simulink model "MassSpringDamper_Simulink_Model"  (R2023b)
settings: Solver=ode45  StartTime=0.0  StopTime=30  MaxStep=0.01  RelTol=1e-3  EnableMultiTasking=on
model workspace (MAT data in the model file):
  c = 1
  k = 2
  m = 3
settings Model: Creator=The MathWorks, Inc.  LastModifiedBy=AmitW
settings SolverCC: AlgebraicLoopSolver=TrustRegion
settings DataIOCC: LimitDataPoints=on  SaveFormat=Array  SaveOutput=off  SignalLogging=off  SaveTime=off  ReturnWorkspaceOutputs=off
settings OptimizationCC: LifeSpan=inf
settings DebuggingCC: UnconnectedInputMsg=warning  UnconnectedOutputMsg=warning  UnconnectedLineMsg=warning  AllowSymbolicDim=off  SFUnexpectedBacktrackingDiag=warning  SFNoUnconditionalDefaultTransitionDiag=warning  SFExecutionAtInitializationDiag=none  ArithmeticOperatorsInVariantConditions=warning
settings HardwareCC: ProdBitPerPointer=32  ProdBitPerSizeT=32  ProdBitPerPtrDiffT=32  ProdLargestAtomicFloat=None  ProdIntDivRoundTo=Undefined  ProdEndianess=Unspecified  ProdWordSize=32  ProdHWDeviceType=32-bit Generic
settings ModelReferenceCC: EnableRefExpFcnMdlSchedulingChecks=on  ModelReferenceMinAlgLoopOccurrences=on  PropagateSignalLabelsOutOfModel=off
settings SFSimCC: SimUseLocalCustomCode=off  CustomCodeUndefinedFunction=UseInterfaceOnly
settings RTWCC: RTWUseLocalCustomCode=off  DLArmComputeVersion=19.05
settings CodeAppCC: StateflowObjectComments=on
settings GRTTargetCC: TargetLangStandard=C89/C90 (ANSI)
settings ConfigComp: CovMetricSettings=dw  CovSaveCumulativeToWorkspaceVar=on  CovSaveSingleToWorkspaceVar=on  CovExternalEMLEnable=off

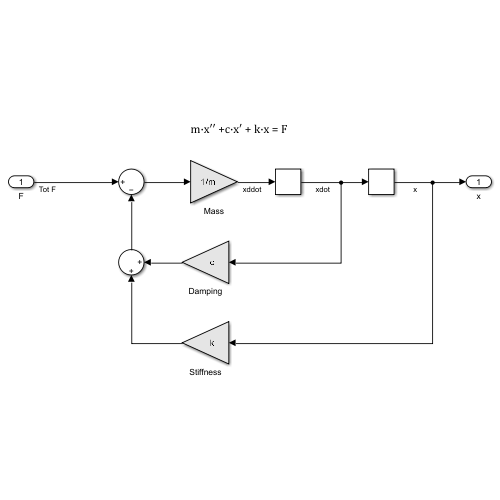
[thumbnail: Simulink's stored preview of the top-level diagram]
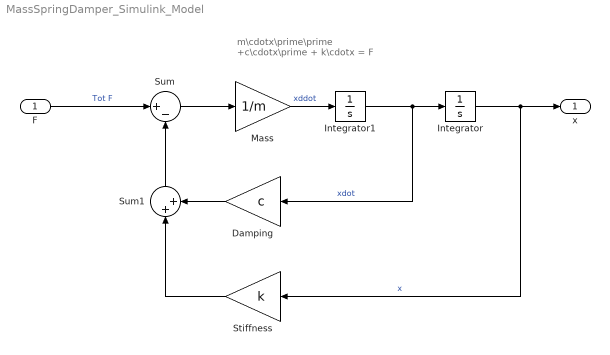
== system MassSpringDamper_Simulink_Model ==
  note: m\cdotx\prime\prime +c\cdotx\prime + k\cdotx = F
  F : Inport  OutDataTypeStr=double  PortDimensions=1  SampleTime=0
  Damping : Gain  SCDEnableBlockLinearizationSpecification=on  Gain=c
  Integrator : Integrator
  Integrator1 : Integrator
  Mass : Gain  SCDEnableBlockLinearizationSpecification=on  Gain=1/m
  Stiffness : Gain  SCDEnableBlockLinearizationSpecification=on  Gain=k
  Sum : Sum  Inputs=|+-
  Sum1 : Sum  Inputs=|++
  x : Outport  OutDataTypeStr=double  PortDimensions=1  SampleTime=0
  wires:
  Integrator1/1 -> Damping/1, Integrator/1  "xdot"
  Damping/1 -> Sum1/2
  Sum/1 -> Mass/1
  Stiffness/1 -> Sum1/1
  F/1 -> Sum/1  "Tot F"
  Mass/1 -> Integrator1/1  "xddot"
  Integrator/1 -> x/1, Stiffness/1  "x"
  Sum1/1 -> Sum/2
